simulink model "E_ZH_Z1"  (R2025a)
settings: Solver=VariableStepAuto  StartTime=0.0  StopTime=10.0  RelTol=1e-3
libraries: ZH_Z x1
settings Model: Creator=Szalay  LastModifiedBy=Szalay
settings RTWCC: RTWVerbose=off

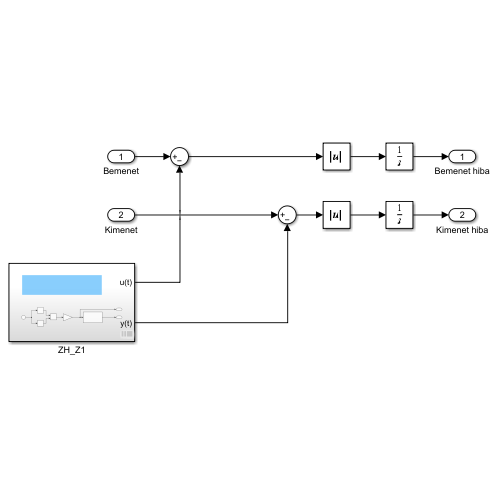
[thumbnail: Simulink's stored preview of the top-level diagram]
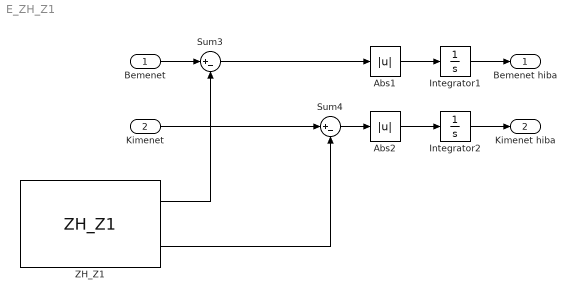
== system E_ZH_Z1 ==
  Bemenet : Inport  OutDataTypeStr=double  PortDimensions=1
  Kimenet : Inport  Port=2  OutDataTypeStr=double  PortDimensions=1
  Abs1 : Abs  SaturateOnIntegerOverflow=off
  Abs2 : Abs  SaturateOnIntegerOverflow=off
  Integrator1 : Integrator
  Integrator2 : Integrator
  Sum3 : Sum  Inputs=|+-
  Sum4 : Sum  Inputs=|+-
  ZH_Z1 : ZH_Z/ZH_Z1  SystemSampleTime=-1  VariantActivationTime=update diagram  EmptyChoice=off  PassThrough=off  PassThroughVariantControl=(default)  EmptyChoiceVariantControl=(default)  AllowFlexibleInterface=on  Latency=0  AutoFrameSizeCalculation=off
  Bemenet hiba : Outport  OutDataTypeStr=double  PortDimensions=1  SampleTime=0
  Kimenet hiba : Outport  Port=2  OutDataTypeStr=double  PortDimensions=1  SampleTime=0
  wires:
  Integrator1/1 -> Bemenet hiba/1
  Bemenet/1 -> Sum3/1
  Abs2/1 -> Integrator2/1
  Integrator2/1 -> Kimenet hiba/1
  Sum3/1 -> Abs1/1
  ZH_Z1/2 -> Sum4/2
  Sum4/1 -> Abs2/1
  ZH_Z1/1 -> Sum3/2
  Kimenet/1 -> Sum4/1
  Abs1/1 -> Integrator1/1
